simulink model "InnerTransitiontoHistoryJunction"  (R2020b)
settings: Solver=VariableStepAuto  StartTime=0.0  StopTime=10.0  RelTol=1e-3
settings Model: Creator=apple  LastModifiedBy=apple

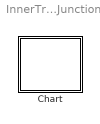
== system InnerTransitiontoHistoryJunction ==
  Chart : Stateflow chart  TreatAsAtomicUnit=on

== stateflow chart InnerTransitiontoHistoryJunction/Chart ==
  note: InnerTransitiontoJunction.thy
  state A
    en:fprintf("Entry A");
    du:fprintf("During A");
    ex:fprintf("Exit A");
    state A1
      en:fprintf("Entry A1");
      du:fprintf("During A1");
      ex:fprintf("Exit A1");
    state A2
      en:fprintf("Entry A2");
      du:fprintf("During A2");
      ex:fprintf("Exit A2");
    A -> (history) : E_one
    (default) -> A1
    A1 -> A2 : E_one
  (default) -> A
  events: E_one local FUNCTION_CALL_EVENT
